simulink model "RocketPowerSim"  (R2025a)
settings: Solver=VariableStepAuto  StartTime=0.0  StopTime=t_end  FixedStep=0.0005  RelTol=1e-3
PreLoadFcn:
  | Constants
values from neighbouring files (symbols this model uses):
  A_ref = pi*r^2    (= 0.00342119439976)    [Constants.m]
  CG = [0; 0; CG_z]    [Constants.m]
  Cl_delta = 0.1    [Constants.m]
  Cn_alpha = 8.0    (= 8)    [Constants.m]
  CP = [0; 0; CP_rocket_z]    [Constants.m]
  d = 0.066    [Constants.m]
  delta_max = delta_max_deg*D2R    (= 0.261799387799)    [Constants.m]
  delta_min = -delta_max    (= -0.261799387799)    [Constants.m]
  g = 9.81    [Constants.m]
  Ixx = 0.0338    [Constants.m]
  Iyy = 0.0338    [Constants.m]
  Izz = 0.001    [Constants.m]
  Kd_pitch = 0.015    [Constants.m]
  Kd_roll = 0.015    [Constants.m]
  Kd_yaw = 0.005    [Constants.m]
  Ki_pitch = 0    [Constants.m]
  Ki_roll = 0    [Constants.m]
  Ki_yaw = 0    [Constants.m]
  Kp_pitch = 0.01    [Constants.m]
  Kp_roll = 0.01    [Constants.m]
  Kp_yaw = 0    [Constants.m]
  L_arm_pitch = L_arm_roll    (= 0.306)    [Constants.m]
  L_arm_roll = CP_fin_z - CG_z    (= 0.306)    [Constants.m]
  L_arm_yaw = r + 0.45*fin_span    (= 0.05235)    [Constants.m]
  m_total = 0.743    [Constants.m]
libraries: simulink_extras x8, slpidlib x3, aerolibutil x2, aerolibanim x1, aerolibadyn x1, aerolibatmos2 x1, aerolibasang x1
settings Model: Creator=alger  LastModifiedBy=alger
settings DataIOCC: ReturnWorkspaceOutputs=off

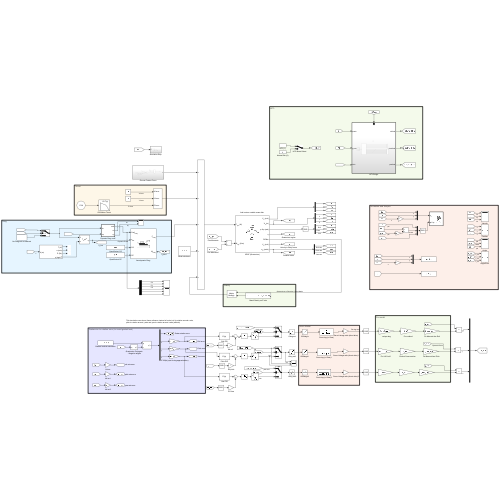
[thumbnail: Simulink's stored preview of the top-level diagram]
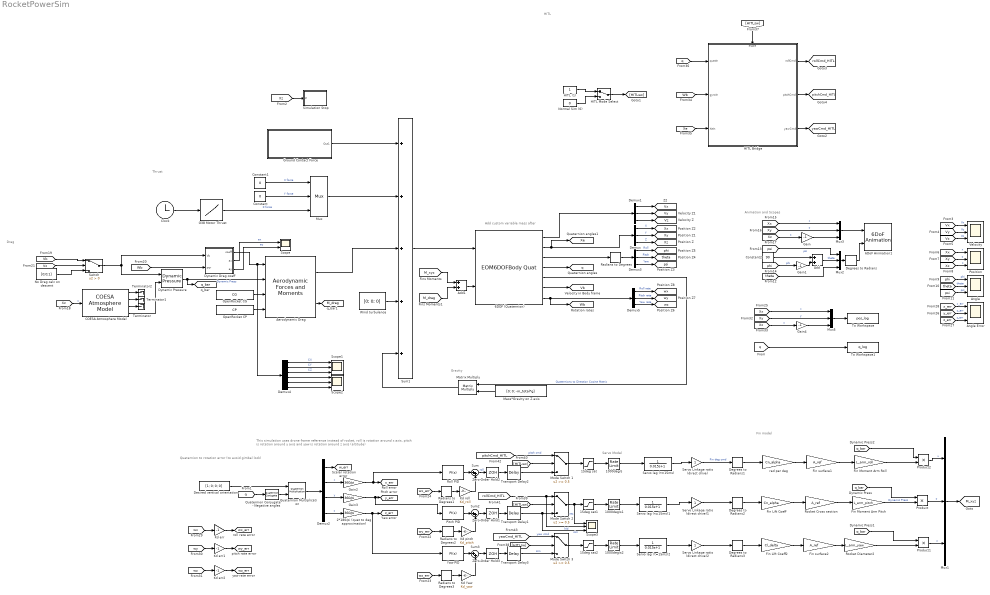
== system RocketPowerSim ==
  note: HITL
  note: Animation and Scopes
  note: Fin model
  note: Servo Model
  note: This simulation uses drone frame reference instead of rocket, roll is rotation around x axis, pitch is rotation around y axis and yaw is rotation around z axis (altitude)
  note: Quaternion to rotation error (to avoid gimbal lock)
  note: Gravity
  note: Thrust
  note: Add custom variable mass after
  note: Drag
  1000deg/s : RateLimiter  RisingSlewLimit=1000  FallingSlewLimit=-1000  SampleTimeMode=inherited
  1000deg/s1 : RateLimiter  RisingSlewLimit=1000  FallingSlewLimit=-1000  SampleTimeMode=inherited
  1000deg/s2 : RateLimiter  RisingSlewLimit=1000  FallingSlewLimit=-1000  SampleTimeMode=inherited
  15deg sat : Saturate  UpperLimit=15  LowerLimit=-15
  15deg sat1 : Saturate  UpperLimit=15  LowerLimit=-15
  15deg sat2 : Saturate  UpperLimit=15  LowerLimit=-15
  2*180/pi (quat to deg approximation) : Gain  Gain=360/pi
  6DOF (Quaternion) : EOM6DOFBodyQuat  eul_0=[0.4 0.4 0]  mass_0=m_total  inertia=[Ixx 0 0; 0 Iyy 0; 0 0 Izz]
  6DoF Animation1 : aerolibanim/6DoF Animation  u1=[-100 100 -100 100 -500 0]  u2=0.1  u3=25  u4=[0 0 0]  u5=Fixed position  u6=[150 150 -50]  u7=20  u8=off
  Add : Sum
  Add1 : Sum
  "Aerodynamic Drag " : aerolibadyn/Aerodynamic Forces and Moments   inputAxes=Body  outputForceAxes=Body  outputMomentAxes=Body  S=pi*(d/2)^2  b=d  cbar=d
  Angle : Scope  NumInputPorts=3
      settings: ActiveDisplayYMinimum=-224.9057193362431  ActiveDisplayYMaximum=224.96947161704185  DataLoggingVariableName=ScopeData2
  Angle Error : Scope  NumInputPorts=3
      settings: ActiveDisplayYMinimum=-25.674641690399241  ActiveDisplayYMaximum=7.95150042092863  DataLoggingVariableName=ScopeData7
  COESA Atmosphere Model : aerolibatmos2/COESA Atmosphere Model  units=Metric (MKS)  spec=1976 COESA-extended U.S. Standard Atmosphere  model=Profile  profile_var=High temperature  profile_percent=1%  profile_alt=5 km (16404 ft)  envelope_var=High temperature  envelope_percent=1%  action=Warning
  Clock : Clock
  Constant : Constant  Value=0
  Constant1 : Constant  Value=0
  Constant2 : Constant  Value=90
  Degrees to Radians{,1..3} (4 alike) : simulink_extras/Transformations/Degrees to Radians
  Demux{,1,3,5} (4 alike) : Demux  Outputs=3
  Demux2 : Demux
  Demux4 : Demux  Outputs=6
  Desired vertical orientation : Constant  Value=[1; 0; 0; 0]
  Dynamic Drag coeff : MATLAB Function  TreatAsAtomicUnit=on
  Dynamic Pressure : aerolibasang/Dynamic Pressure
  Fin Lift Coeff : Gain  Gain=Cn_alpha
  Fin Lift Coeff2 : Gain  Gain=Cl_delta
  Fin Moment Arm Pitch : Gain  Gain=L_arm_pitch
  Fin Moment Arm Roll : Gain  Gain=L_arm_roll
  Fin surface1 : Gain  Gain=A_ref
  Fin surface2 : Gain  Gain=A_ref
  G38 Motor Thrust : Lookup_n-D  NumberOfTableDimensions=1  BreakpointsForDimension1=[0, 0.024, 0.171, 0.497, 1.0, 1.279, 1.498, 1.783, 2.011, 2.272, 2.467, 2.64]  Table=[0, 52.928, 48.424, 45.045, 42.23, 39.978, 36.599, 30.406, 23.086, 10.135, 3.941, 0]  ExtrapMethod=Clip  InternalRulePriority=Speed  RndMeth=Simplest
  Gain : Gain  Gain=-1
  Gain1 : Gain  Gain=-1
  Gain2 : Gain  Gain=360/pi
  Gain3 : Gain  Gain=360/pi
  Gain4 : Gain  Gain=-1
  Ground Contact Force : Subsystem
  HITL (1) : Constant
  HITL Bridge : Subsystem  TreatAsAtomicUnit=on
  HITL Mode Select : ManualSwitch
  Kd Yaw : Gain  Gain=Kd_yaw
  Kd err : Gain  Gain=-1
  Kd err1 : Gain  Gain=-1
  Kd err2 : Gain  Gain=-1
  Kd pitch : Gain  Gain=Kd_pitch
  Kd roll : Gain  Gain=Kd_roll
  Mass*Gravity on Z axis : Constant  Value=[0; 0; -m_total*g]
  Matrix Multiply : Product  Multiplication=Matrix(*)
  Mode Switch 1 : Switch  Threshold=0.5  SaturateOnIntegerOverflow=off  InputSameDT=off
  Mode Switch 2 : Switch  Threshold=0.5  SaturateOnIntegerOverflow=off  InputSameDT=off
  Mode Switch 3 : Switch  Threshold=0.5  SaturateOnIntegerOverflow=off  InputSameDT=off
  Mux{,1..3,5} (5 alike) : Mux  Inputs=3
      Mux settings: DisplayOption=signals
  No Drag calc on descent : Constant  Value=[0;0;1]
  Normal Sim (0) : Constant  Value=0
  OpenRocket CG : Constant  Value=CG
  OpenRocket CP : Constant  Value=CP
  Pitch PID : slpidlib/PID Controller  Controller=PI  Form=Parallel  TimeDomain=Continuous-time  UseExternalTs=off  SampleTime=-1  IntegratorMethod=Forward Euler  FilterMethod=Forward Euler  ControllerParametersSource=internal  P=Kp_pitch  I=Ki_pitch  UseKiTs=off  D=0  UseExternalDerivativeSource=off  N=10  UseFilter=on  TunerSelectOption=Transfer Function Based (PID Tuner App)  InitialConditionSource=internal  InitialConditionForIntegrator=0  InitialConditionForFilter=0  DifferentiatorICPrevScaledInput=0  ExternalReset=none  TrackingMode=off  Kt=1  LimitOutput=off  SatLimitsSource=internal  UpperSaturationLimit=delta_max  LowerSaturationLimit=delta_min  LinearizeAsGain=on  AntiWindupMode=back-calculation  Kb=1  LimitIntegrator=off  UpperIntegratorSaturationLimit=inf  LowerIntegratorSaturationLimit=-inf  POutMin=[]  POutMax=[]  IOutMin=[]  IOutMax=[]  DOutMin=[]  DOutMax=[]  NOutMin=[]  NOutMax=[]  SumOutMin=[]  SumOutMax=[]  SaturationOutMin=[]  SaturationOutMax=[]  PParamMin=[]  PParamMax=[]  IParamMin=[]  IParamMax=[]  DParamMin=[]  DParamMax=[]  NParamMin=[]  NParamMax=[]  KbParamMin=[]  KbParamMax=[]  KtParamMin=[]  KtParamMax=[]  KbOutMin=[]  KbOutMax=[]  KtOutMin=[]  KtOutMax=[]  IntegratorOutMin=[]  IntegratorOutMax=[]  FilterOutMin=[]  FilterOutMax=[]  SumI1OutMin=[]  SumI1OutMax=[]  SumI2OutMin=[]  SumI2OutMax=[]  SumI3OutMin=[]  SumI3OutMax=[]  SumI4OutMin=[]  SumI4OutMax=[]  SumDOutMin=[]  SumDOutMax=[]  DifferentiatorOutMin=[]  DifferentiatorOutMax=[]  FilterDiffOutCoefMin=[]  FilterDiffOutCoefMax=[]  ReciprocalOutMin=[]  ReciprocalOutMax=[]  SumDenOutMin=[]  SumDenOutMax=[]  SumNumOutMin=[]  SumNumOutMax=[]  DivideOutMin=[]  DivideOutMax=[]  UdiffTsProdOutMin=[]  UdiffTsProdOutMax=[]  NTsProdOutMin=[]  NTsProdOutMax=[]  UintegralTsProdOutMin=[]  UintegralTsProdOutMax=[]  UngainTsProdOutMin=[]  UngainTsProdOutMax=[]  ClampingZeroOutDataTypeStr=Inherit: Inherit via back propagation  ClampingZeroOutMin=[]  ClampingZeroOutMax=[]  FilterDenConstantOutDataTypeStr=Inherit: Inherit via back propagation  FilterDenConstantOutMin=[]  FilterDenConstantOutMax=[]  PCopyOutDataTypeStr=Inherit: Inherit via back propagation  PCopyOutMin=[]  PCopyOutMax=[]  NCopyOutDataTypeStr=Inherit: Inherit via back propagation  NCopyOutMin=[]  NCopyOutMax=[]  IntegratorContinuousStateAttributes=''  IntegratorStateMustResolveToSignalObject=off  IntegratorRTWStateStorageClass=Auto  FilterContinuousStateAttributes=''  FilterStateMustResolveToSignalObject=off  FilterRTWStateStorageClass=Auto  ParallelPVariant=InternalParameters  IdealPVariant=Disabled  IVariant=InternalParameters  DVariant=Disabled  IntegratorVariant=Continuous  SatVariant=Disabled  AWVariant=Passthrough  PCopyVariant=Disabled  TRVariant=Disabled  FdbkBlocksVariant=Forward  IdealPFdbkVariant=Disabled  SatFdbkVariant=Disabled  DerivativeFilterVariant=Disabled  NVariant=Disabled  NCopyVariant=Disabled_SignalSpec  FilterICVariant=Disabled  IntegratorICVariant=InternalICs  ExternalResetVariant=Disabled  TRSumVariant=Passthrough  SumFdbkVariant=Disabled  SumVariant=Sum_PI  TsampFilterVariant=InternalTs  TsampNgainVariant=Passthrough  TsampIntegralVariant=Disabled_SignalSpec  ExternalSaturationOutDataTypeStr=Inherit: Same as second input  DerivativeSourceVariant=Disabled  PreIntVariant=InternalPreInt
  Position : Scope  NumInputPorts=3
      settings: ActiveDisplayYMinimum=-212.5671132286864  ActiveDisplayYMaximum=289.6805654056418
  Product : Product
  Product1 : Product
  Product2 : Product
  Quaternion Multiplication : aerolibutil/Quaternion Multiplication
  Quaternion Conjugate - Negative angles : aerolibutil/Quaternion Conjugate
  Radians to Degrees{,1..3} (4 alike) : simulink_extras/Transformations/Radians to Degrees
  Rocket Cross section : Gain  Gain=A_ref
  Rocket Diameter2 : Gain  Gain=L_arm_yaw
  Roll PID : slpidlib/PID Controller  Controller=PI  Form=Parallel  TimeDomain=Continuous-time  UseExternalTs=off  SampleTime=-1  IntegratorMethod=Forward Euler  FilterMethod=Forward Euler  ControllerParametersSource=internal  P=Kp_roll  I=Ki_roll  UseKiTs=off  D=0  UseExternalDerivativeSource=off  N=10  UseFilter=on  TunerSelectOption=Transfer Function Based (PID Tuner App)  InitialConditionSource=internal  InitialConditionForIntegrator=0  InitialConditionForFilter=0  DifferentiatorICPrevScaledInput=0  ExternalReset=none  TrackingMode=off  Kt=1  LimitOutput=off  SatLimitsSource=internal  UpperSaturationLimit=delta_max  LowerSaturationLimit=delta_min  LinearizeAsGain=on  AntiWindupMode=back-calculation  Kb=1  LimitIntegrator=off  UpperIntegratorSaturationLimit=inf  LowerIntegratorSaturationLimit=-inf  POutMin=[]  POutMax=[]  IOutMin=[]  IOutMax=[]  DOutMin=[]  DOutMax=[]  NOutMin=[]  NOutMax=[]  SumOutMin=[]  SumOutMax=[]  SaturationOutMin=[]  SaturationOutMax=[]  PParamMin=[]  PParamMax=[]  IParamMin=[]  IParamMax=[]  DParamMin=[]  DParamMax=[]  NParamMin=[]  NParamMax=[]  KbParamMin=[]  KbParamMax=[]  KtParamMin=[]  KtParamMax=[]  KbOutMin=[]  KbOutMax=[]  KtOutMin=[]  KtOutMax=[]  IntegratorOutMin=[]  IntegratorOutMax=[]  FilterOutMin=[]  FilterOutMax=[]  SumI1OutMin=[]  SumI1OutMax=[]  SumI2OutMin=[]  SumI2OutMax=[]  SumI3OutMin=[]  SumI3OutMax=[]  SumI4OutMin=[]  SumI4OutMax=[]  SumDOutMin=[]  SumDOutMax=[]  DifferentiatorOutMin=[]  DifferentiatorOutMax=[]  FilterDiffOutCoefMin=[]  FilterDiffOutCoefMax=[]  ReciprocalOutMin=[]  ReciprocalOutMax=[]  SumDenOutMin=[]  SumDenOutMax=[]  SumNumOutMin=[]  SumNumOutMax=[]  DivideOutMin=[]  DivideOutMax=[]  UdiffTsProdOutMin=[]  UdiffTsProdOutMax=[]  NTsProdOutMin=[]  NTsProdOutMax=[]  UintegralTsProdOutMin=[]  UintegralTsProdOutMax=[]  UngainTsProdOutMin=[]  UngainTsProdOutMax=[]  ClampingZeroOutDataTypeStr=Inherit: Inherit via back propagation  ClampingZeroOutMin=[]  ClampingZeroOutMax=[]  FilterDenConstantOutDataTypeStr=Inherit: Inherit via back propagation  FilterDenConstantOutMin=[]  FilterDenConstantOutMax=[]  PCopyOutDataTypeStr=Inherit: Inherit via back propagation  PCopyOutMin=[]  PCopyOutMax=[]  NCopyOutDataTypeStr=Inherit: Inherit via back propagation  NCopyOutMin=[]  NCopyOutMax=[]  IntegratorContinuousStateAttributes=''  IntegratorStateMustResolveToSignalObject=off  IntegratorRTWStateStorageClass=Auto  FilterContinuousStateAttributes=''  FilterStateMustResolveToSignalObject=off  FilterRTWStateStorageClass=Auto  ParallelPVariant=InternalParameters  IdealPVariant=Disabled  IVariant=InternalParameters  DVariant=Disabled  IntegratorVariant=Continuous  SatVariant=Disabled  AWVariant=Passthrough  PCopyVariant=Disabled  TRVariant=Disabled  FdbkBlocksVariant=Forward  IdealPFdbkVariant=Disabled  SatFdbkVariant=Disabled  DerivativeFilterVariant=Disabled  NVariant=Disabled  NCopyVariant=Disabled_SignalSpec  FilterICVariant=Disabled  IntegratorICVariant=InternalICs  ExternalResetVariant=Disabled  TRSumVariant=Passthrough  SumFdbkVariant=Disabled  SumVariant=Sum_PI  TsampFilterVariant=InternalTs  TsampNgainVariant=Passthrough  TsampIntegralVariant=Disabled_SignalSpec  ExternalSaturationOutDataTypeStr=Inherit: Same as second input  DerivativeSourceVariant=Disabled  PreIntVariant=InternalPreInt
  Scope : Scope  NumInputPorts=2
      settings: ActiveDisplayYMinimum=-3.9269209431036742  ActiveDisplayYMaximum=3.926946267229888  DataLoggingVariableName=ScopeData3
  Scope1 : Scope  NumInputPorts=3
      settings: ActiveDisplayYMinimum=-1.920796326794896  ActiveDisplayYMaximum=13.287166941154068  DataLoggingVariableName=ScopeData4
  Scope2 : Scope  NumInputPorts=3
      settings: ActiveDisplayYMinimum=-1.920796326794896  ActiveDisplayYMaximum=13.287166941154068  DataLoggingVariableName=ScopeData5
  Scope3 : Scope  NumInputPorts=3
      settings: ActiveDisplayYMinimum=-266.9159049987793  ActiveDisplayYMaximum=280.7528190612793  DataLoggingVariableName=ScopeData6
  Servo Linkage ratio (direct drive) : Gain
  Servo Linkage ratio (direct drive)1 : Gain
  Servo Linkage ratio (direct drive)2 : Gain
  Servo lag (τ=15ms) : TransferFcn  Denominator=[0.015 1]
  Servo lag (τ=15ms)1 : TransferFcn  Denominator=[0.015 1]
  Servo lag (τ=15ms)2 : TransferFcn  Denominator=[0.015 1]
  Simulation Stop : Subsystem
  Sum : Sum  Inputs=|++
  Sum1 : Sum  Inputs=+++++
  Sum2 : Sum  Inputs=|++
  Sum3 : Sum  Inputs=|++
  Switch : Switch  Criteria=u2 > Threshold  SaturateOnIntegerOverflow=off  InputSameDT=off
  Terminator : Terminator
  Terminator1 : Terminator
  Terminator2 : Terminator
  To Workspace : ToWorkspace  VariableName=pos_log  SampleTime=-1
  To Workspace1 : ToWorkspace  VariableName=q_log  SampleTime=-1
  Transport Delay1 : TransportDelay  DelayTime=0.015
  Transport Delay2 : TransportDelay  DelayTime=0.015
  Transport Delay3 : TransportDelay  DelayTime=0.015
  Velocity : Scope  NumInputPorts=3
      settings: ActiveDisplayYMinimum=-98.301975894653125  ActiveDisplayYMaximum=100.74131931342991
  Wind turbulence : Constant  Value=[0; 0; 0]
  Yaw PID : slpidlib/PID Controller  Controller=PI  Form=Parallel  TimeDomain=Continuous-time  UseExternalTs=off  SampleTime=-1  IntegratorMethod=Forward Euler  FilterMethod=Forward Euler  ControllerParametersSource=internal  P=Kp_yaw  I=Ki_yaw  UseKiTs=off  D=0  UseExternalDerivativeSource=off  N=10  UseFilter=on  TunerSelectOption=Transfer Function Based (PID Tuner App)  InitialConditionSource=internal  InitialConditionForIntegrator=0  InitialConditionForFilter=0  DifferentiatorICPrevScaledInput=0  ExternalReset=none  TrackingMode=off  Kt=1  LimitOutput=off  SatLimitsSource=internal  UpperSaturationLimit=delta_max  LowerSaturationLimit=delta_min  LinearizeAsGain=on  AntiWindupMode=back-calculation  Kb=1  LimitIntegrator=off  UpperIntegratorSaturationLimit=inf  LowerIntegratorSaturationLimit=-inf  POutMin=[]  POutMax=[]  IOutMin=[]  IOutMax=[]  DOutMin=[]  DOutMax=[]  NOutMin=[]  NOutMax=[]  SumOutMin=[]  SumOutMax=[]  SaturationOutMin=[]  SaturationOutMax=[]  PParamMin=[]  PParamMax=[]  IParamMin=[]  IParamMax=[]  DParamMin=[]  DParamMax=[]  NParamMin=[]  NParamMax=[]  KbParamMin=[]  KbParamMax=[]  KtParamMin=[]  KtParamMax=[]  KbOutMin=[]  KbOutMax=[]  KtOutMin=[]  KtOutMax=[]  IntegratorOutMin=[]  IntegratorOutMax=[]  FilterOutMin=[]  FilterOutMax=[]  SumI1OutMin=[]  SumI1OutMax=[]  SumI2OutMin=[]  SumI2OutMax=[]  SumI3OutMin=[]  SumI3OutMax=[]  SumI4OutMin=[]  SumI4OutMax=[]  SumDOutMin=[]  SumDOutMax=[]  DifferentiatorOutMin=[]  DifferentiatorOutMax=[]  FilterDiffOutCoefMin=[]  FilterDiffOutCoefMax=[]  ReciprocalOutMin=[]  ReciprocalOutMax=[]  SumDenOutMin=[]  SumDenOutMax=[]  SumNumOutMin=[]  SumNumOutMax=[]  DivideOutMin=[]  DivideOutMax=[]  UdiffTsProdOutMin=[]  UdiffTsProdOutMax=[]  NTsProdOutMin=[]  NTsProdOutMax=[]  UintegralTsProdOutMin=[]  UintegralTsProdOutMax=[]  UngainTsProdOutMin=[]  UngainTsProdOutMax=[]  ClampingZeroOutDataTypeStr=Inherit: Inherit via back propagation  ClampingZeroOutMin=[]  ClampingZeroOutMax=[]  FilterDenConstantOutDataTypeStr=Inherit: Inherit via back propagation  FilterDenConstantOutMin=[]  FilterDenConstantOutMax=[]  PCopyOutDataTypeStr=Inherit: Inherit via back propagation  PCopyOutMin=[]  PCopyOutMax=[]  NCopyOutDataTypeStr=Inherit: Inherit via back propagation  NCopyOutMin=[]  NCopyOutMax=[]  IntegratorContinuousStateAttributes=''  IntegratorStateMustResolveToSignalObject=off  IntegratorRTWStateStorageClass=Auto  FilterContinuousStateAttributes=''  FilterStateMustResolveToSignalObject=off  FilterRTWStateStorageClass=Auto  ParallelPVariant=InternalParameters  IdealPVariant=Disabled  IVariant=InternalParameters  DVariant=Disabled  IntegratorVariant=Continuous  SatVariant=Disabled  AWVariant=Passthrough  PCopyVariant=Disabled  TRVariant=Disabled  FdbkBlocksVariant=Forward  IdealPFdbkVariant=Disabled  SatFdbkVariant=Disabled  DerivativeFilterVariant=Disabled  NVariant=Disabled  NCopyVariant=Disabled_SignalSpec  FilterICVariant=Disabled  IntegratorICVariant=InternalICs  ExternalResetVariant=Disabled  TRSumVariant=Passthrough  SumFdbkVariant=Disabled  SumVariant=Sum_PI  TsampFilterVariant=InternalTs  TsampNgainVariant=Passthrough  TsampIntegralVariant=Disabled_SignalSpec  ExternalSaturationOutDataTypeStr=Inherit: Same as second input  DerivativeSourceVariant=Disabled  PreIntVariant=InternalPreInt
  Zero-Order Hold1 : ZeroOrderHold  SampleTime=0.02
  Zero-Order Hold2 : ZeroOrderHold  SampleTime=0.02
  Zero-Order Hold3 : ZeroOrderHold  SampleTime=0.02
  rad per deg : Gain  Gain=Cn_alpha
  tag scope: M_drag=global, M_xyz=global, Vb=global, Vx=global, Vy=global, Vz=global, Wb=global, Xe=global, Xx=global, Xy=global, Xz=global, phi=global, pitchCmd_HITL=global, psi=global, q=global, q_bar=global, rollCmd_HITL=global, theta=global, w_err=global, wx=global, wx_err=global, wy=global, wy_err=global, wz=global, wz_err=global, x_err=global, y_err=global, yawCmd_HITL=global, z_err=global
  wires:
  Clock/1 -> G38 Motor Thrust/1
  G38 Motor Thrust/1 -> Mux/3  "Z force"
  Constant/1 -> Mux/2  "Y force"
  Constant1/1 -> Mux/1  "X force"
  6DOF (Quaternion)/4 -> [q]
  Mass*Gravity on Z axis/1 -> Matrix Multiply/2
  6DOF (Quaternion)/2 -> Demux/1, [Xe]
  Demux/3 -> [Xz]  "Z"
  Demux1/3 -> [Vz]
  Demux1/2 -> [Vy]
  Demux1/1 -> [Vx]
  6DOF (Quaternion)/1 -> Demux1/1
  Dynamic Drag coeff/1(coeff) -> Demux4/1, "Aerodynamic Drag "/1
  Dynamic Pressure/1 -> [q_bar], "Aerodynamic Drag "/2  "Dynamic Press"
  OpenRocket CG/1 -> "Aerodynamic Drag "/3
  OpenRocket CP/1 -> "Aerodynamic Drag "/4
  6DOF (Quaternion)/5 -> Matrix Multiply/1  "Quaternions to Direction Cosine Matrix"
  [q] -> Quaternion Conjugate - Negative angles/1
  Quaternion Multiplication/1 -> Demux2/1
  Demux2/1 -> [w_err]
  Demux2/3 -> Gain3/1  "y"
  Desired vertical orientation/1 -> Quaternion Multiplication/1
  Quaternion Conjugate - Negative angles/1 -> Quaternion Multiplication/2
  Fin Lift Coeff/1 -> Rocket Cross section/1
  Rocket Cross section/1 -> Fin Moment Arm Pitch/1
  Fin Moment Arm Pitch/1 -> Product/2
  [q_bar] -> Product/1  "Dynamic Press"
  [q_bar] -> Product1/1
  Product1/1 -> Mux1/3  "z"
  Product/1 -> Mux1/2  "y"
  Mux1/1 -> [M_xyz]
  [Xz] -> Simulation Stop/1(Z)
  Demux/2 -> [Xy]  "Y"
  Demux/1 -> [Xx]  "X"
  6DOF (Quaternion)/3 -> Radians to Degrees/1
  Demux3/1 -> [phi]  "Roll"
  Demux3/3 -> [psi]  "Yaw"
  [Vx] -> Velocity/1  "Vx"
  [Vy] -> Velocity/2  "Vy"
  [Vz] -> Velocity/3  "Vz"
  [Xz] -> Position/3  "z"
  [Xy] -> Position/2  "y"
  [Xx] -> Position/1  "x"
  [phi] -> Angle/1  "phi"
  [theta] -> Angle/2  "theta"
  [psi] -> Angle/3  "psi"
  Radians to Degrees/1 -> Demux3/1
  Product2/1 -> Mux1/1  "x"
  [q_bar] -> Product2/1
  Demux2/2 -> Gain2/1  "x"
  6DOF (Quaternion)/6 -> [Vb]
  Fin Moment Arm Roll/1 -> Product2/2
  Fin surface1/1 -> Fin Moment Arm Roll/1
  rad per deg/1 -> Fin surface1/1
  Fin surface2/1 -> Rocket Diameter2/1
  Fin Lift Coeff2/1 -> Fin surface2/1
  Demux2/4 -> 2*180/pi (quat to deg approximation)/1  "z"
  Rocket Diameter2/1 -> Product1/2
  Mux/1 -> Sum1/2
  Sum1/1 -> 6DOF (Quaternion)/1
  Matrix Multiply/1 -> Sum1/5
  Ground Contact Force/1(Out1) -> Sum1/1
  [theta] -> Mux2/3
  [Xx] -> Mux3/1  "x"
  Degrees to Radians/1 -> 6DoF Animation1/2
  Gain/1 -> Mux3/3
  [phi] -> Gain1/1  "phi"
  Mux3/1 -> 6DoF Animation1/1
  Gain1/1 -> Add/2
  Add/1 -> Mux2/2  "theta"
  Mux2/1 -> Degrees to Radians/1
  [Xy] -> Mux3/2  "y"
  [Xz] -> Gain/1  "z"
  [psi] -> Mux2/1  "psi"
  Constant2/1 -> Add/1
  [Xz] -> COESA Atmosphere Model/1  "z"
  COESA Atmosphere Model/4 -> Dynamic Pressure/2
  COESA Atmosphere Model/3 -> Terminator/1
  COESA Atmosphere Model/2 -> Terminator1/1
  COESA Atmosphere Model/1 -> Terminator2/1
  Switch/1 -> Dynamic Pressure/1, Dynamic Drag coeff/1(Vb)
  6DOF (Quaternion)/7 -> Demux5/1, [Wb]
  [Wb] -> Dynamic Drag coeff/2(pqr)
  Dynamic Drag coeff/2(ax) -> Scope/1  "ax"
  Dynamic Drag coeff/3(ay) -> Scope/2  "ay"
  [Vz] -> Switch/2
  [Vb] -> Switch/1
  No Drag calc on descent/1 -> Switch/3
  Demux4/1 -> Scope1/1  "CX"
  Demux4/2 -> Scope1/2  "CY"
  Demux4/3 -> Scope1/3  "CZ"
  Demux4/4 -> Scope2/1
  Demux4/5 -> Scope2/2
  Demux4/6 -> Scope2/3
  Roll PID/1 -> Sum/1
  Yaw PID/1 -> Sum3/1
  Pitch PID/1 -> Sum2/1
  [wy_err] -> Radians to Degrees2/1
  [wz_err] -> Radians to Degrees3/1
  [wx_err] -> Radians to Degrees1/1
  Kd roll/1 -> Sum/2
  Kd pitch/1 -> Sum2/2
  Kd Yaw/1 -> Sum3/2
  Gain2/1 -> [x_err], Roll PID/1
  Gain3/1 -> Pitch PID/1, [y_err]
  2*180/pi (quat to deg approximation)/1 -> [z_err], Yaw PID/1
  15deg sat1/1 -> 1000deg/s1/1
  15deg sat2/1 -> 1000deg/s2/1
  1000deg/s/1 -> Servo lag (τ=15ms)/1
  Servo lag (τ=15ms)1/1 -> Servo Linkage ratio (direct drive)1/1
  1000deg/s1/1 -> Servo lag (τ=15ms)1/1
  Servo lag (τ=15ms)2/1 -> Servo Linkage ratio (direct drive)2/1
  1000deg/s2/1 -> Servo lag (τ=15ms)2/1
  Servo Linkage ratio (direct drive)/1 -> Degrees to Radians1/1  "Fin deg cmd"
  Servo Linkage ratio (direct drive)1/1 -> Degrees to Radians2/1
  Servo Linkage ratio (direct drive)2/1 -> Degrees to Radians3/1
  Demux5/3 -> [wz]  "Yaw rate"
  Demux5/2 -> [wy]  "Pitch rate"
  Demux5/1 -> [wx]  "Roll rate"
  Degrees to Radians1/1 -> rad per deg/1
  Degrees to Radians2/1 -> Fin Lift Coeff/1
  Degrees to Radians3/1 -> Fin Lift Coeff2/1
  Demux3/2 -> [theta]  "Pitch"
  Servo lag (τ=15ms)/1 -> Servo Linkage ratio (direct drive)/1
  15deg sat/1 -> 1000deg/s/1
  "Aerodynamic Drag "/1 -> Sum1/3
  Wind turbulence/1 -> Sum1/4
  [M_xyz] -> Add1/1
  Add1/1 -> 6DOF (Quaternion)/2
  Radians to Degrees1/1 -> Kd roll/1
  [z_err] -> Angle Error/3  "z_err"
  [y_err] -> Angle Error/2  "y_err"
  [x_err] -> Angle Error/1  "x_err"
  [wx] -> Kd err/1
  Kd err/1 -> [wx_err]
  Kd err1/1 -> [wy_err]
  [wy] -> Kd err1/1
  [wz] -> Kd err2/1
  Kd err2/1 -> [wz_err]
  Radians to Degrees2/1 -> Kd pitch/1
  Radians to Degrees3/1 -> Kd Yaw/1
  [Xx] -> Mux5/1  "x"
  [Xz] -> Gain4/1  "z"
  [Xy] -> Mux5/2  "y"
  Mux5/1 -> To Workspace/1
  [q] -> To Workspace1/1
  Gain4/1 -> Mux5/3
  "Aerodynamic Drag "/2 -> [M_drag]
  [M_drag] -> Add1/2
  HITL (1)/1 -> HITL Mode Select/1
  Normal Sim (0)/1 -> HITL Mode Select/2
  Sum/1 -> Zero-Order Hold2/1  "roll"
  Mode Switch 1/1 -> 15deg sat/1
  Mode Switch 2/1 -> Scope3/1, 15deg sat1/1  "res"
  Sum3/1 -> Zero-Order Hold3/1
  Mode Switch 3/1 -> 15deg sat2/1
  [Wb] -> HITL Bridge/2(gyroIn)
  [Xe] -> HITL Bridge/3(XeIn)
  [q] -> HITL Bridge/1(quatIn)
  HITL Mode Select/1 -> [HITLsw]
  [HITLsw] -> HITL Bridge/Enable
  [HITLsw] -> Mode Switch 3/2
  [HITLsw] -> Mode Switch 2/2
  [HITLsw] -> Mode Switch 1/2
  HITL Bridge/1(rollCmd) -> [rollCmd_HITL]
  HITL Bridge/2(pitchCmd) -> [pitchCmd_HITL]
  HITL Bridge/3(yawCmd) -> [yawCmd_HITL]
  [rollCmd_HITL] -> Scope3/2, Mode Switch 2/1  "hitl"
  [pitchCmd_HITL] -> Mode Switch 1/1  "pitch cmd"
  Zero-Order Hold2/1 -> Transport Delay2/1
  Transport Delay2/1 -> Mode Switch 1/3
  Sum2/1 -> Zero-Order Hold1/1
  Zero-Order Hold1/1 -> Transport Delay1/1
  [yawCmd_HITL] -> Mode Switch 3/1  "yaw cmd"
  Transport Delay1/1 -> Scope3/3, Mode Switch 2/3  "sim"
  Zero-Order Hold3/1 -> Transport Delay3/1
  Transport Delay3/1 -> Mode Switch 3/3  "sim"

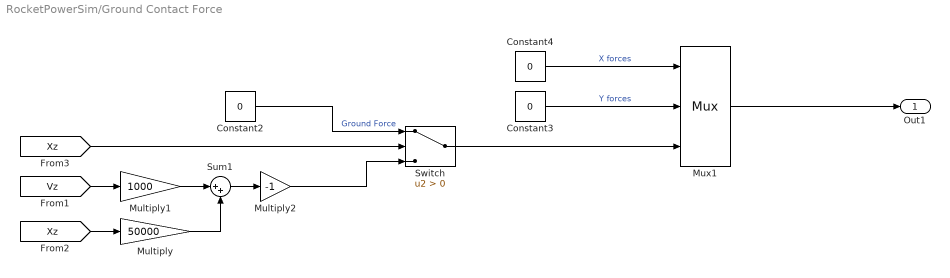
== system RocketPowerSim/Ground Contact Force ==
  Constant2 : Constant  Value=0
  Constant3 : Constant  Value=0
  Constant4 : Constant  Value=0
  Multiply : Gain  Gain=50000
  Multiply1 : Gain  Gain=1000
  Multiply2 : Gain  Gain=-1
  Mux1 : Mux  Inputs=3
      settings: DisplayOption=signals
  Sum1 : Sum  Inputs=|++
  Switch : Switch  Criteria=u2 > Threshold  SaturateOnIntegerOverflow=off  InputSameDT=off
  Out1 : Outport
  wires:
  Constant4/1 -> Mux1/1  "X forces"
  [Xz] -> Multiply/1
  [Xz] -> Switch/2
  Constant3/1 -> Mux1/2  "Y forces"
  [Vz] -> Multiply1/1
  Sum1/1 -> Multiply2/1
  Switch/1 -> Mux1/3
  Multiply2/1 -> Switch/3
  Multiply1/1 -> Sum1/1
  Multiply/1 -> Sum1/2
  Mux1/1 -> Out1/1
  Constant2/1 -> Switch/1  "Ground Force"

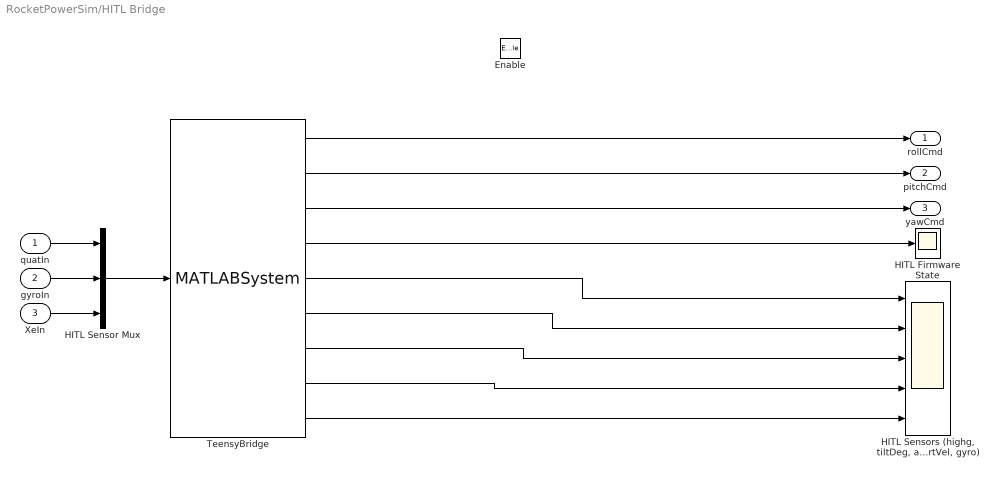
== system RocketPowerSim/HITL Bridge ==
  quatIn : Inport
  gyroIn : Inport  Port=2
  XeIn : Inport  Port=3
  Enable : EnablePort
  HITL Firmware State : Scope
  HITL Sensor Mux : Mux  Inputs=3
  "HITL Sensors (highg, tiltDeg, altitude, vertVel, gyro)" : Scope  NumInputPorts=5
  TeensyBridge : MATLABSystem  System=TeensyBridge  ComPort=COM16  BaudRate=115200  Ts=0.01  ResponseTimeoutS=0.5  SimulateUsing=Interpreted execution
      mask Type: TeensyBridge
  rollCmd : Outport
  pitchCmd : Outport  Port=2
  yawCmd : Outport  Port=3
  wires:
  quatIn/1 -> HITL Sensor Mux/1
  gyroIn/1 -> HITL Sensor Mux/2
  XeIn/1 -> HITL Sensor Mux/3
  HITL Sensor Mux/1 -> TeensyBridge/1
  TeensyBridge/1 -> rollCmd/1
  TeensyBridge/4 -> HITL Firmware State/1
  TeensyBridge/5 -> "HITL Sensors (highg, tiltDeg, altitude, vertVel, gyro)"/1
  TeensyBridge/6 -> "HITL Sensors (highg, tiltDeg, altitude, vertVel, gyro)"/2
  TeensyBridge/7 -> "HITL Sensors (highg, tiltDeg, altitude, vertVel, gyro)"/3
  TeensyBridge/8 -> "HITL Sensors (highg, tiltDeg, altitude, vertVel, gyro)"/4
  TeensyBridge/9 -> "HITL Sensors (highg, tiltDeg, altitude, vertVel, gyro)"/5
  TeensyBridge/2 -> pitchCmd/1
  TeensyBridge/3 -> yawCmd/1

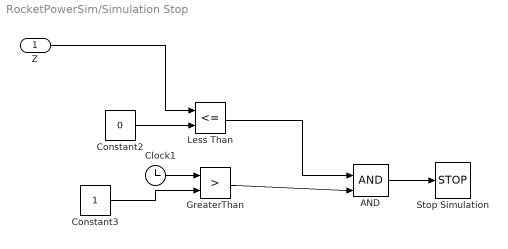
== system RocketPowerSim/Simulation Stop ==
  Z : Inport
  AND : Logic  IconShape=distinctive  AllPortsSameDT=off  OutDataTypeStr=boolean
  Clock1 : Clock
  Constant2 : Constant  Value=0
  Constant3 : Constant
  GreaterThan : RelationalOperator  Operator=>  OutDataTypeStr=boolean  RndMeth=Simplest  InputSameDT=off
  Less Than : RelationalOperator  Operator=<=  OutDataTypeStr=boolean  RndMeth=Simplest  InputSameDT=off
  Stop Simulation : Stop
  wires:
  Less Than/1 -> AND/1
  AND/1 -> Stop Simulation/1
  Constant3/1 -> GreaterThan/2
  Constant2/1 -> Less Than/2
  GreaterThan/1 -> AND/2
  Z/1 -> Less Than/1
  Clock1/1 -> GreaterThan/1

== matlab function RocketPowerSim/Dynamic Drag coeff ==
  data: Vb input; coeff output; pqr input; ax output; ay output
function [coeff, ax, ay] = fcn(Vb, pqr)
%FCN  Aerodynamic coefficients, axisymmetric rocket, body +z = nose/thrust.
%
% Inputs:
%   Vb  : [u; v; w] velocity in BODY axes [m/s] (air-relative if wind exists)
%   pqr : [p; q; r] body rates about x, y, z [rad/s]
% Outputs:
%   coeff : [Cx Cy Cz Cl Cm Cn], scaled downstream by the aero block as
%           F = qbar*S*C, M = qbar*S*d*C  (S, d in block dialog must match)
%   ax,ay : incidence angles [rad] — angle between the body z-axis and
%           the VELOCITY vector (not attitude).
%
% Model: linear derivatives, valid to ~10-15 deg incidence, forward
% flight only (w > 0). The external apogee latch must zero the aero at
% w = 0 — past that point ax/ay sit on the atan2 branch cut.

  %% Constants -------------------------------------------------------------
  CA0 = 0.4;   % [-]     axial drag coeff at zero incidence (Mach table later)
  CNa = 8;     % [1/rad] normal-force slope, whole rocket. Reconciled with
               %         Constants.m's Cn_alpha (was 2.0, disagreed -- see
               %         its comment). Still not a real OpenRocket/wind-
               %         tunnel value, just no longer two different guesses.
  SM  = 1.33;  % [cal]   static margin, CP behind CG (shifts during burn)
  d   = 0.066; % [m]     reference diameter, must equal aero block setting
  Cmq = -20;   % [-]     pitch damping (tilt about y). STILL A PLACEHOLDER --
               %         tried computing this properly (Barrowman strip
               %         theory), got a number 10x this one, but found a
               %         real fin-count ambiguity in that derivation AND a
               %         deeper question of whether the linear form used
               %         here is even the right model (OpenRocket's own
               %         thesis uses a quadratic-in-rate drag-based model
               %         for this specific term instead). Left as-is rather
               %         than replace one guess with a shakier one.
  Clp = -20;   % [-]     roll damping  (tilt about x), = Cmq by symmetry.
               %         Same caveat as Cmq above.
  Cnr = -6.58; % [-]     spin damping about the long axis. [COMPUTED] via
               %         Barrowman roll-damping formula (RocketPy docs /
               %         OpenRocket thesis eq 3.69), trapezoidal-fin closed
               %         form, using (CNa)_1 = CNa/n_fins = 2.0/rad as a
               %         per-fin approximation (not a real per-fin
               %         OpenRocket component-analysis value yet -- pull
               %         that to refine this further). Was -5 placeholder,
               %         close to this computed value -- good sanity check.

  %% Flow state ------------------------------------------------------------
  Vs = max(norm(Vb), 0.1);      % airspeed, floored: no div-by-zero on pad

  ax = atan2(Vb(1), Vb(3));     % velocity lean toward body x [rad]
  ay = atan2(Vb(2), Vb(3));     % velocity lean toward body y [rad]

  ci = Vb(3)/Vs;                % cos(incidence): axial fraction of the
                                % flow, ~1 in normal flight. Makes Cz
                                % respond to tilt instead of sitting
                                % frozen at -CA0.

  %% Coefficients ----------------------------------------------------------
  coeff = zeros(1, 6);          % explicit size for Coder

  % Forces: lateral push opposing the tilt; axial drag scaled by the
  % axial flow fraction.
  coeff(1) = -CNa*ax;                            % Cx
  coeff(2) = -CNa*ay;                            % Cy
  coeff(3) = -CA0*ci;                            % Cz

  % Moments: weathercock spring (lateral force at CP, lever arm SM
  % calibers) + rate damper (pqr nondimensionalized by d/(2*Vs)).
  % Cl/Cm sign difference falls out of the cross product, not physics.
  coeff(4) = -CNa*SM*ay + Clp*pqr(1)*d/(2*Vs);   % Cl (tilt about x)
  coeff(5) =  CNa*SM*ax + Cmq*pqr(2)*d/(2*Vs);   % Cm (tilt about y)
  coeff(6) =  Cnr*pqr(3)*d/(2*Vs);               % Cn (spin: damper only)
end
